simulink model "ABS_Model"  (R2020b)
settings: Solver=ode45  StartTime=0.0  StopTime=50  MaxStep=0.01  RelTol=1e-3  AbsTol=1e-6
PreLoadFcn:
  | abs_data;
undefined symbols (not defined in the file): g, m, mu, Rr, sigbuilder_block, slip, v0
settings Model: OrderedModelArguments=off  Creator=ADMIN  LastModifiedBy=ADMIN
settings DebuggingCC: AlgebraicLoopMsg=none

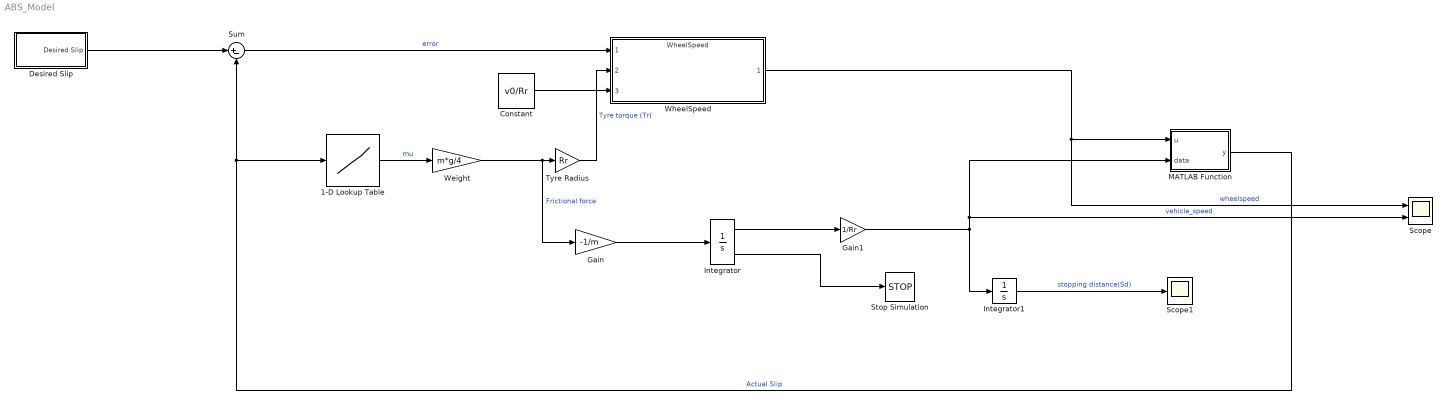
== system ABS_Model ==
  1-D Lookup Table : Lookup_n-D  NumberOfTableDimensions=1  BreakpointsForDimension1=slip  Table=mu  InternalRulePriority=Speed  RndMeth=Simplest  InputSameDT=on
  Constant : Constant  Value=v0/Rr
  Desired Slip : Subsystem  Tag=STV Subsys  LoadFcn=sigbuilder_block('load');  StartFcn=sigbuilder_block('start');  StopFcn=sigbuilder_block('stop');  ClipboardFcn=sigbuilder_block('clipboard');  mask(Sigbuilder block){tuvar=[0:10]}
      mask help: Simulink:masks:SigbuilderBlock_MD
      mask init:
      | if ~strcmp(get_param(bdroot(gcbh),'SimulationStatus'),'stopped') tuvar = sigbuilder_block('maskInit'); end
      settings: CopyFcn=sigbuilder_block('copy');  DeleteFcn=sigbuilder_block('delete');  ModelCloseFcn=sigbuilder_block('modelClose');  PreSaveFcn=sigbuilder_block('preSave');  PauseFcn=sigbuilder_block('pause');  ContinueFcn=sigbuilder_block('continue');  NameChangeFcn=sigbuilder_block('namechange');  OpenFcn=sigbuilder_block('open',[437.6 199.2 550.4 400 ]);  CloseFcn=sigbuilder_block('close');
      mask Display: plot(0, 0, 100, 100,[2, 2, 32, 32, 2], [68, 8, 8, 68, 68],[32, 2], [38, 38], [32, 19, 2],[53, 60, 44], [32, 17, 17, 2],[16, 16, 31, 31]);txt = getActiveGroup(gcbh);text(2, 100, txt,'verticalAlignment', 'top');
  Gain : Gain  Gain=-1/m
  Gain1 : Gain  Gain=1/Rr
  Integrator : Integrator  InitialCondition=v0  LimitOutput=on  UpperSaturationLimit=1000  LowerSaturationLimit=0  ShowSaturationPort=on
  Integrator1 : Integrator
  MATLAB Function : MATLAB Function  TreatAsAtomicUnit=on
  Scope : Scope  NumInputPorts=2
  Scope1 : Scope
  Stop Simulation : Stop
  Sum : Sum  Inputs=|+-
  Tyre Radius : Gain  Gain=Rr
  Weight : Gain  Gain=m*g/4
  WheelSpeed : ModelReference  ModelNameDialog=WheelSpeed  ModelReferenceVersion=1.17
  wires:
  1-D Lookup Table/1 -> Weight/1  "mu"
  Weight/1 -> Gain/1, Tyre Radius/1  "Frictional force"
  Tyre Radius/1 -> WheelSpeed/2  "Tyre torque (Tr)"
  WheelSpeed/1 -> MATLAB Function/1(u), Scope/1  "wheelspeed"
  Integrator/1 -> Gain1/1
  Integrator1/1 -> Scope1/1  "stopping distance(Sd)"
  Integrator/2 -> Stop Simulation/1
  Constant/1 -> WheelSpeed/3
  Gain/1 -> Integrator/1
  Gain1/1 -> Scope/2, MATLAB Function/2(data), Integrator1/1  "vehicle_speed"
  Desired Slip/1(Desired Slip) -> Sum/1
  Sum/1 -> WheelSpeed/1  "error"
  MATLAB Function/1(y) -> Sum/2, 1-D Lookup Table/1  "Actual Slip"

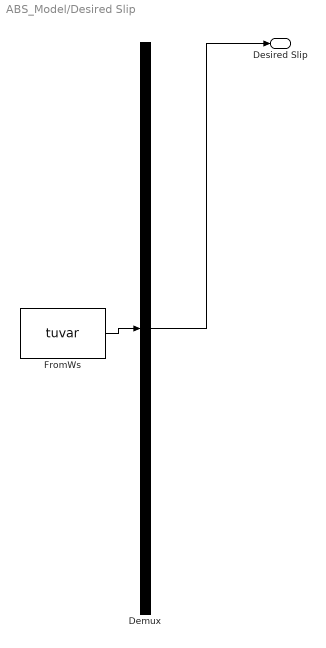
== system ABS_Model/Desired Slip ==
  Demux : Demux  Tag=STV Demux  Outputs=1
      settings: DisplayOption=none
  FromWs : FromWorkspace  Tag=STV FromWs  VariableName=tuvar
      SigBuilderData=|
      | common.afterFinalStr = 'Extrapolate'
      | common.sampleTime = 0
      | dataSet.timeRange = [0 50]
      | dataSet.name = 'Group 1'
      | sbobj.Groups.Name = 'Group 1'
      | sbobj.Groups.Signals.Name = 'Desired Slip'
      | sbobj.Groups.Signals.XData = [0 50]
      | sbobj.Groups.Signals.YData = [0.2 0.2]
      | sbobj.Groups.TimeRange = [0 50]
  Desired Slip : Outport  Tag=STV Outport
  wires:
  FromWs/1 -> Demux/1
  Demux/1 -> Desired Slip/1

== matlab function ABS_Model/MATLAB Function ==
  data: u input; y output; data input
function y = slip(u, data)

y = 1-(u/(data + (data==0)*eps));
